simulink model "train_simulink"  (R2015a)
settings: Solver=ode45  StartTime=0.0  StopTime=10.0  RelTol=1e-3
libraries: slctrlblks x1, simulink x1
settings Model: Creator=gabrielle  LastModifiedBy=gabrielle

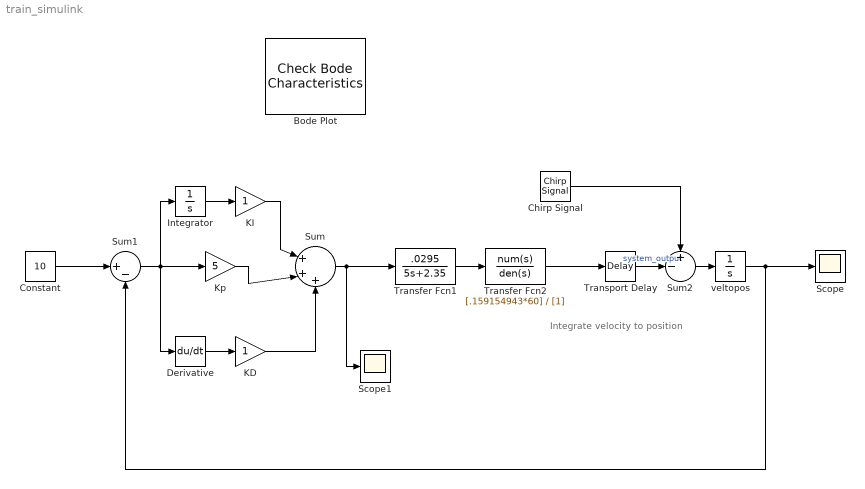
== system train_simulink ==
  note: Integrate velocity to position
  Bode Plot : slctrlblks/Model Verification/Check Bode  Characteristics  InstantiateOnLoad=on  SaveOperatingPoints=off  LinearizationIOs={'/Sum', 1, 'in', 'on', '';'/Sum2', 1, 'out', 'on', ''}  LinearizeAt=SnapshotTimes  SnapshotTimes=[0]  TriggerType=rising  SampleTime=auto  RateConversionMethod=zoh  PreWarpFreq=10  UseExactDelayModel=off  UseFullBlockNameLabels=off  UseBusSignalLabels=off  enabled=on  stopWhenAssertionFail=off  export=off  ViewDlgPos=[]  OpenViewOnLoad=off  LaunchViewOnOpen=on  FrequencyUnits=rad/s  MagnitudeUnits=dB  PhaseUnits=deg  TimeUnits=seconds  EnableUpperBound=off  UpperBoundFrequencies=[]  UpperBoundMagnitudes=[]  EnableLowerBound=off  LowerBoundFrequencies=[]  LowerBoundMagnitudes=[]
  Chirp Signal : simulink/Sources/Chirp Signal  f1=0.1  T=100  f2=.8
  Constant : Constant  Value=10
  Derivative : Derivative
  Integrator : Integrator
  KD : Gain
  KI : Gain
  Kp : Gain  Gain=5
  Scope : Scope
  Scope1 : Scope
  Sum : Sum  Inputs=|+++
  Sum1 : Sum  Inputs=|+-
  Sum2 : Sum  Inputs=+-|
  Transfer Fcn1 : TransferFcn  Numerator=[.0295]  Denominator=[5 2.35]
  Transfer Fcn2 : TransferFcn  Numerator=[.159154943*60]  Denominator=[1]
  Transport Delay : TransportDelay
  "veltopos " : Integrator
  wires:
  Integrator/1 -> KI/1
  Derivative/1 -> KD/1
  KD/1 -> Sum/3
  Sum1/1 -> Derivative/1, Integrator/1, Kp/1
  Constant/1 -> Sum1/1
  Kp/1 -> Sum/2
  KI/1 -> Sum/1
  Sum/1 -> Transfer Fcn1/1, Scope1/1
  "veltopos "/1 -> Scope/1, Sum1/2
  Chirp Signal/1 -> Sum2/1
  Transport Delay/1 -> Sum2/2  "system_output"
  Sum2/1 -> "veltopos "/1
  Transfer Fcn1/1 -> Transfer Fcn2/1
  Transfer Fcn2/1 -> Transport Delay/1
